simulink model "SimConnectToolboxExample"  (R2020b)
settings: Solver=FixedStepDiscrete  StartTime=0.0  StopTime=inf  FixedStep=0.03  RelTol=1e-3
libraries: SimConnectToolbox x3
settings Model: EnablePacing=on  Creator=Andreas  LastModifiedBy=Andreas
settings DebuggingCC: InheritedTsInSrcMsg=none

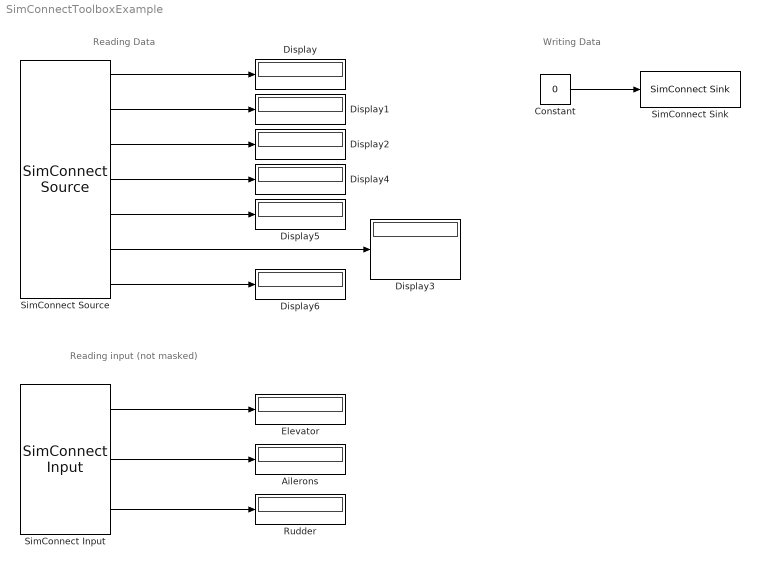
== system SimConnectToolboxExample ==
  note: Reading input (not masked)
  note: Reading Data
  note: Writing Data
  Ailerons : Display
  Constant : Constant  Value=0
  Display{,1..6} (7 alike) : Display
  Elevator : Display
  Rudder : Display
  SimConnect Input : SimConnectToolbox/SimConnect Input  configurationIndex=0  connectionName=SimConnectInput  variables=|
      | AXIS_ELEVATOR_SET, FALSE;
      | AXIS_AILERONS_SET, FALSE;
      | AXIS_RUDDER_SET, FALSE;
      settings: SourceProductName=SimConnect Toolbox
      mask Display:
      | % This is a new mask on top of the base mask.
      | % Use "View base mask" link below to see the base mask.
      | port_label('output', 1, '\delta_\eta', 'texmode', 'on')
      | port_label('output', 2, '\delta_\xi', 'texmode', 'on')
      | port_label('output', 3, '\delta_\zeta', 'texmode', 'on')
  SimConnect Sink : SimConnectToolbox/SimConnect Sink  configurationIndex=0  connectionName=SimConnectSink  variables=RUDDER TRIM PCT, Percent Over 100;
      settings: SourceProductName=SimConnect Toolbox
      mask Display:
      | % This is a new mask on top of the base mask.
      | % Use "View base mask" link below to see the base mask.
      | port_label('input', 1, 'Rudder Trim', 'texmode', 'on')
  SimConnect Source : SimConnectToolbox/SimConnect Source  configurationIndex=0  connectionName=SimConnectSource  variables=|
      | G FORCE, GFORCE;
      | PLANE PITCH DEGREES, RADIANS;
      | PLANE BANK DEGREES, RADIANS;
      | AIRSPEED INDICATED, KNOTS;
      | PLANE ALTITUDE, FEET;
      | STRUCT WORLD ROTATION VELOCITY, STRUCT;
      | LIGHT STROBE ON, BOOL;
      settings: SourceProductName=SimConnect Toolbox
      mask Display:
      | % This is a new mask on top of the base mask.
      | % Use "View base mask" link below to see the base mask.
      | port_label('output', 1, 'g', 'texmode', 'on')
      | port_label('output', 2, '\Theta (rad)', 'texmode', 'on')
      | port_label('output', 3, '\Phi (rad)', 'texmode', 'on')
      | port_label('output', 4, 'IAS (kts)', 'texmode', 'on')
      | port_label('output', 5, 'Alt (ft)', 'texmode', 'on')
      | port_label('output', 6, 'World R-Velocity', 'texmode', 'on')
      | port_label('output', 7, 'Strobe-Light On', 'texmode', 'on')
  wires:
  Constant/1 -> SimConnect Sink/1
  SimConnect Source/1 -> Display/1
  SimConnect Source/2 -> Display1/1
  SimConnect Source/3 -> Display2/1
  SimConnect Source/6 -> Display3/1
  SimConnect Input/1 -> Elevator/1
  SimConnect Input/2 -> Ailerons/1
  SimConnect Input/3 -> Rudder/1
  SimConnect Source/4 -> Display4/1
  SimConnect Source/5 -> Display5/1
  SimConnect Source/7 -> Display6/1
